simulink model "Airshow_hotpursuit_traning_timer"  (R2012b)
settings: Solver=ode45  StartTime=0.0  StopTime=inf  RelTol=1e-3
libraries: dspswit3 x5
settings Model: Creator=airshow  LastModifiedBy=airshow

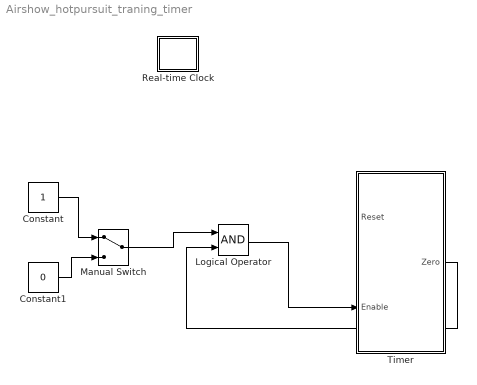
== system Airshow_hotpursuit_traning_timer ==
  Constant : Constant
  Constant1 : Constant  Value=0
  Logical Operator : Logic  AllPortsSameDT=off  OutDataTypeStr=boolean
  Manual Switch : ManualSwitch
  Real-time Clock : Subsystem  mask(Real-time Clock){sample_time=0.02, tolerance=1}
      mask prompts: sample_time "Synchronize with real-time every n seconds:"; tolerance "Real-time warning tolerance (seconds):"
      mask help: Real-time Synchronization Block
      mask Help: This block synchronizes simulation time with the PC real-time clock or UNIX system clock. The first dialog entry is the period at which the clock is checked to insure real-time synchronization. The second dialog entry is the number of seconds that the simulation time must be within real-time before a warning is printed.
      mask Display: plot(0,0,100,100,[40,60,60,54,54,64,69,76,82,77,81,83,83,81,78,74,70,64,57,49,41,35,32,30,30,31,34,40,47,47,40,40],[90,90,85,85,80,79,76,87,80,70,64,57,49,41,33,28,24,22,21,23,25,31,37,46,56,65,73,78,80,85,85,90],[69,53,53],[64,50,73])
  Timer : Subsystem
  wires:
  Timer/1(Zero) -> Logical Operator/2
  Logical Operator/1 -> Timer/2(Enable)
  Constant/1 -> Manual Switch/1
  Constant1/1 -> Manual Switch/2
  Manual Switch/1 -> Logical Operator/1

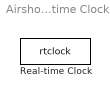
== system Airshow_hotpursuit_traning_timer/Real-time Clock ==
  Real-time Clock : S-Function  FunctionName=rtclock  Parameters=sample_time, tolerance  EnableBusSupport=off

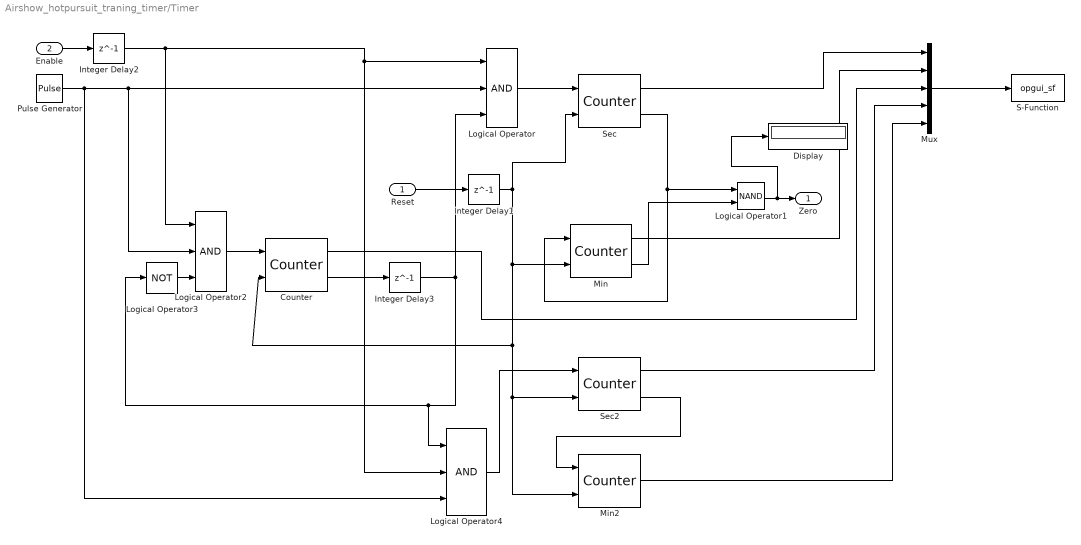
== system Airshow_hotpursuit_traning_timer/Timer ==
  Reset : Inport
  Enable : Inport  Port=2
  Counter : dspswit3/Counter  Direction=Down  CountEvent=Falling edge  CounterSize=User defined  MaxCount=4  InitialCount=4  Output=Count and Hit  HitValue=0  ResetInput=on  SamplesPerFrame=1  Ts=1  CntDtype=double  HitDtype=Boolean
  Display : Display
  Integer Delay1 : Delay  DelayLength=1
  Integer Delay2 : Delay  DelayLength=1
  Integer Delay3 : Delay  DelayLength=1
  Logical Operator : Logic  Inputs=3  AllPortsSameDT=off  OutDataTypeStr=boolean
  Logical Operator1 : Logic  Operator=NAND  AllPortsSameDT=off  OutDataTypeStr=boolean
  Logical Operator2 : Logic  Inputs=3  AllPortsSameDT=off  OutDataTypeStr=boolean
  Logical Operator3 : Logic  Operator=NOT  Inputs=1  AllPortsSameDT=off  OutDataTypeStr=boolean
  Logical Operator4 : Logic  Inputs=3  AllPortsSameDT=off  OutDataTypeStr=boolean
  Min : dspswit3/Counter  Direction=Down  CountEvent=Falling edge  CounterSize=User defined  MaxCount=2  InitialCount=1  Output=Count and Hit  HitValue=0  ResetInput=on  SamplesPerFrame=1  Ts=1  CntDtype=double  HitDtype=Logical
  Min2 : dspswit3/Counter  Direction=Up  CountEvent=Falling edge  CounterSize=User defined  MaxCount=59  InitialCount=0  Output=Count  HitValue=0  ResetInput=on  SamplesPerFrame=1  Ts=1  CntDtype=double  HitDtype=Logical
  Mux : Mux  Inputs=5
  Pulse Generator : DiscretePulseGenerator  SampleTime=0.5
  S-Function : S-Function  FunctionName=opgui_sf  Parameters=0.5  EnableBusSupport=off
  Sec : dspswit3/Counter  Direction=Down  CountEvent=Falling edge  CounterSize=User defined  MaxCount=59  InitialCount=00  Output=Count and Hit  HitValue=0  ResetInput=on  SamplesPerFrame=1  Ts=1  CntDtype=double  HitDtype=Logical
  Sec2 : dspswit3/Counter  Direction=Up  CountEvent=Falling edge  CounterSize=User defined  MaxCount=59  InitialCount=0  Output=Count and Hit  HitValue=59  ResetInput=on  SamplesPerFrame=1  Ts=1  CntDtype=double  HitDtype=Logical
  Zero : Outport
  wires:
  Reset/1 -> Integer Delay1/1
  Enable/1 -> Integer Delay2/1
  Logical Operator1/1 -> Display/1, Zero/1
  Mux/1 -> S-Function/1
  Sec/1 -> Mux/1
  Logical Operator/1 -> Sec/1
  Counter/2 -> Integer Delay3/1
  Counter/1 -> Mux/3
  Min/1 -> Mux/2
  Logical Operator2/1 -> Counter/1
  Integer Delay3/1 -> Logical Operator3/1, Logical Operator4/1, Logical Operator/3
  Sec2/2 -> Min2/1
  Logical Operator4/1 -> Sec2/1
  Sec2/1 -> Mux/4
  Min2/1 -> Mux/5
  Integer Delay2/1 -> Logical Operator4/2, Logical Operator/1, Logical Operator2/1
  Pulse Generator/1 -> Logical Operator4/3, Logical Operator/2, Logical Operator2/2
  Logical Operator3/1 -> Logical Operator2/3
  Min/2 -> Logical Operator1/2
  Integer Delay1/1 -> Counter/2, Sec2/2, Min2/2, Min/2, Sec/2
  Sec/2 -> Min/1, Logical Operator1/1
